simulink model "Decision_Planning_Unit"  (R2019a)
settings: Solver=ode2  StartTime=0.0  StopTime=inf  FixedStep=0.002  RelTol=1e-3  EnableMultiTasking=on
undefined symbols (not defined in the file): qc_get_step_size
libraries: simulink x5, quarc_library x1
settings Model: Creator=User  LastModifiedBy=mbohra
settings SolverCC: PositivePriorityOrder=on
settings DataIOCC: ReturnWorkspaceOutputs=off
settings DebuggingCC: PregeneratedLibrarySubsystemCodeDiagnostic=none  ArithmeticOperatorsInVariantConditions=warning
settings SFSimCC: SimUseLocalCustomCode=off
settings RTWCC: SystemTargetFile=quarc_linux_nvidia.tlc  TemplateMakefile=quarc_linux_nvidia_tmf  Description=QUARC Linux Nvidia Target  RTWUseLocalCustomCode=off
settings STFCustomTargetCC: TargetLibSuffix=.a  TargetPreCompLibLocation=C:\PROGRA~3\QUARC\lib\2019a\LINUX_~1\release  TargetLangStandard=C99 (ISO)  ConcurrentExecutionCompliant=on  SystemTargetFile=quarc_linux_nvidia.tlc
settings GRTTargetCC: TargetLibSuffix=.a  TargetPreCompLibLocation=C:\PROGRA~3\QUARC\lib\2019a\LINUX_~1\release  ParMdlRefBuildCompliant=off  CompOptLevelCompliant=off  CombineOutputUpdateFcns=off  MatFileLogging=off  CPPClassGenCompliant=off  GRTInterface=on  UseToolchainInfoCompliant=off  ExtMode=on  ExtModeMexFile=quarc_comm  ExtModeMexArgs='-w -d /tmp -uri %u'

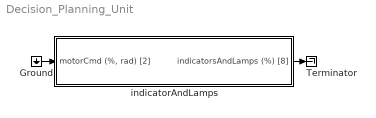
== system Decision_Planning_Unit ==
  Ground : Ground
  Terminator : Terminator
  indicatorAndLamps : Subsystem
  wires:
  Ground/1 -> indicatorAndLamps/1("motorCmd (%, rad) [2]")
  indicatorAndLamps/1(indicatorsAndLamps (%) [8]) -> Terminator/1

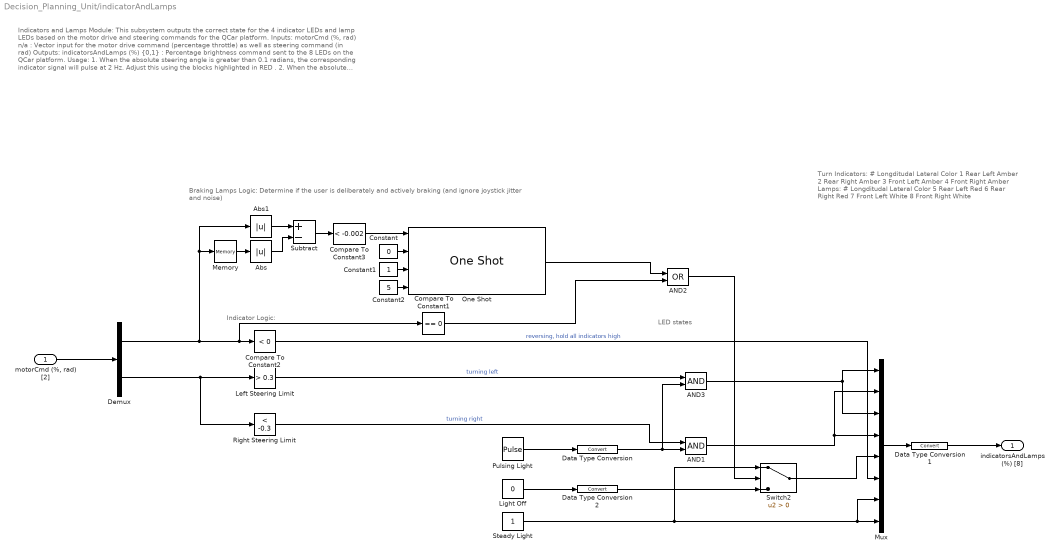
== system Decision_Planning_Unit/indicatorAndLamps ==
  note: Indicator Logic:
  note: Turn Indicators:
      | # Longditudal Lateral Color
      | 1 Rear Left Amber
      | 2 Rear Right Amber
      | 3 Front Left Amber
      | 4 Front Right Amber
      |
      | Lamps:
      | # Longditudal Lateral Color
      | 5 Rear Left Red
      | 6 Rear Right Red
      | 7 Front Left White
      | 8 Front Right White
  note: LED states
  note: Braking Lamps Logic:
      | Determine if the user is deliberately and actively braking (and ignore joystick jitter and noise)
  note: Indicators and Lamps Module:
      |
      | This subsystem outputs the correct state for the 4 indicator LEDs and lamp LEDs based on the motor drive and steering commands for the QCar platform.
      |
      | Inputs:
      | motorCmd (%, rad) n/a : Vector input for the motor drive command (percentage throttle) as well as steering command (in rad)
      |
      | Outputs:
      | indicatorsAndLamps (%) {0,1} : Percentage brightness command sent to the 8 LEDs on the QCar platform.
      |
      | Usage:
      | 1. When the absolute steering angle is greater than 0.1 radians, the corresponding indicator signal will pulse at 2 Hz. Adjust this using the blocks highlighted in RED .
      | 2. When the absolute motor drive command approaches 0, the brake lamps will receive 100% brightness command, and 0% brightness otherwise. Adjust this using the blocks highlighted in GREEN .
  "motorCmd (%, rad) [2]" : Inport
  AND1 : Logic  IconShape=distinctive  AllPortsSameDT=off  OutDataTypeStr=boolean
  AND2 : Logic  Operator=OR  IconShape=distinctive  AllPortsSameDT=off  OutDataTypeStr=boolean
  AND3 : Logic  IconShape=distinctive  AllPortsSameDT=off  OutDataTypeStr=boolean
  Abs : Abs
  Abs1 : Abs
  Compare To Constant1 : simulink/Logic and Bit Operations/Compare To Constant  relop===  const=0  OutDataTypeStr=uint8
  Compare To Constant2 : simulink/Logic and Bit Operations/Compare To Constant  relop=<  const=0  OutDataTypeStr=boolean
  Compare To Constant3 : simulink/Logic and Bit Operations/Compare To Constant  relop=<  const=-0.002  OutDataTypeStr=boolean
  Constant : Constant  Value=0
  Constant1 : Constant
  Constant2 : Constant  Value=5
  Data Type Conversion : DataTypeConversion
  Data Type Conversion1 : DataTypeConversion
  Data Type Conversion2 : DataTypeConversion
  Demux : Demux  Outputs=2
  Left Steering Limit : simulink/Logic and Bit Operations/Compare To Constant  relop=>  const=0.3  OutDataTypeStr=boolean
  Light Off : Constant  Value=0  OutDataTypeStr=boolean
  Memory : Memory
  Mux : Mux  Inputs=8
  One Shot : quarc_library/Discontinuities/One Shot  trigger_type=Falling edge  redun_pulse=Ignore extraneous pulse  width_source=External input port  pulse_width=100
      settings: SourceProductName=QUARC Targets
  Pulsing Light : DiscretePulseGenerator  Period=0.5/qc_get_step_size  PulseWidth=0.5/2/qc_get_step_size  SampleTime=qc_get_step_size
  Right Steering Limit : simulink/Logic and Bit Operations/Compare To Constant  relop=<  const=-0.3  OutDataTypeStr=boolean
  Steady Light : Constant  OutDataTypeStr=boolean
  Subtract : Sum  Inputs=+-
  Switch2 : Switch  Criteria=u2 > Threshold
  indicatorsAndLamps (%) [8] : Outport
  wires:
  AND2/1 -> Switch2/2
  Compare To Constant1/1 -> AND2/2
  Compare To Constant2/1 -> Mux/6  "reversing, hold all indicators high"
  AND1/1 -> Mux/4, Mux/2
  Subtract/1 -> Compare To Constant3/1
  "motorCmd (%, rad) [2]"/1 -> Demux/1
  AND3/1 -> Mux/3, Mux/1
  Demux/1 -> Abs1/1, Memory/1, Compare To Constant2/1, Compare To Constant1/1
  Constant1/1 -> One Shot/3
  Switch2/1 -> Mux/5
  Left Steering Limit/1 -> AND3/1  "turning left"
  Data Type Conversion1/1 -> indicatorsAndLamps (%) [8]/1
  Data Type Conversion/1 -> AND1/2, AND3/2
  Abs1/1 -> Subtract/1
  Memory/1 -> Abs/1
  Abs/1 -> Subtract/2
  Pulsing Light/1 -> Data Type Conversion/1
  Constant/1 -> One Shot/2
  Mux/1 -> Data Type Conversion1/1
  Right Steering Limit/1 -> AND1/1  "turning right"
  Constant2/1 -> One Shot/4
  Compare To Constant3/1 -> One Shot/1
  Steady Light/1 -> Switch2/1, Mux/8, Mux/7
  One Shot/1 -> AND2/1
  Light Off/1 -> Data Type Conversion2/1
  Demux/2 -> Left Steering Limit/1, Right Steering Limit/1
  Data Type Conversion2/1 -> Switch2/3
